simulink model "IntegratedLocalizationProcessor"  (R2023b)
settings: Solver=VariableStepAuto  StartTime=0.0  StopTime=10.0  RelTol=1e-3
undefined symbols (not defined in the file or in its folder): Discrete, fractalcoef, Time
libraries: mspsensorlib x1, ctrlSharedLib x1
settings Model: Creator=user  LastModifiedBy=user

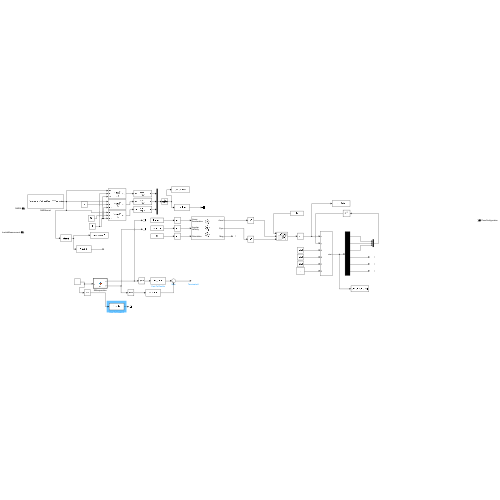
[thumbnail: Simulink's stored preview of the top-level diagram]
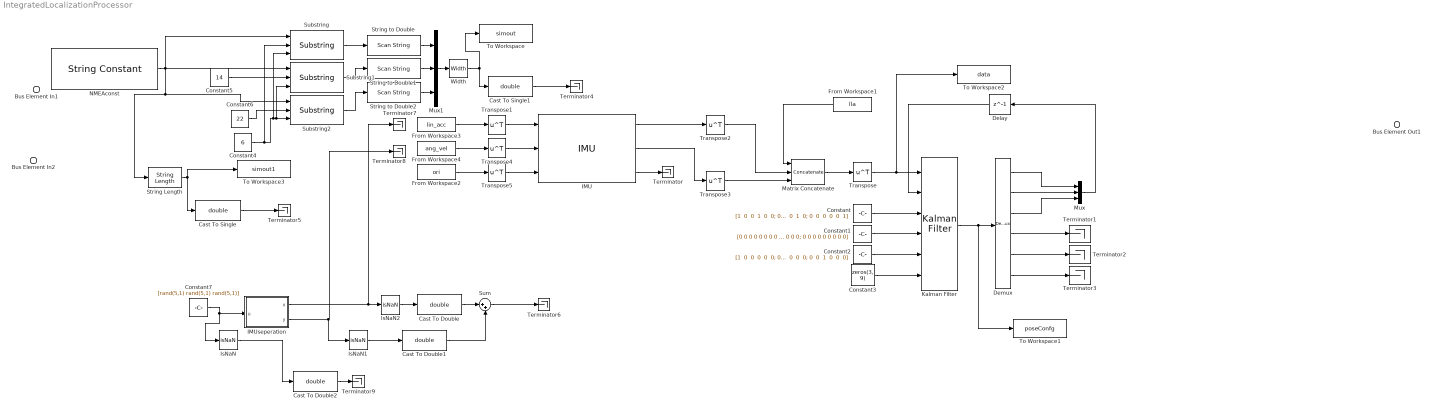
== system IntegratedLocalizationProcessor ==
  Bus Element In1 : Inport  PortName=NMEA
  Bus Element In2 : Inport  Port=2  PortName=InertialMeasurement
  Cast To Double : DataTypeConversion  OutDataTypeStr=double  SaturateOnIntegerOverflow=off  RndMeth=Floor
  Cast To Double1 : DataTypeConversion  OutDataTypeStr=double  SaturateOnIntegerOverflow=off  RndMeth=Floor
  Cast To Double2 : DataTypeConversion  OutDataTypeStr=double  SaturateOnIntegerOverflow=off  RndMeth=Floor
  Cast To Single : DataTypeConversion  OutDataTypeStr=double  SaturateOnIntegerOverflow=off  RndMeth=Floor
  Cast To Single1 : DataTypeConversion  OutDataTypeStr=double  SaturateOnIntegerOverflow=off  RndMeth=Floor
  Constant : Constant  Value=|
      | [1  0  0  1  0  0;
      | 0  1  0  0  1  0;
      | 0  0  1  0  0  1;
      | 0  0  0  1  0  0;
      | 0  0  0  0  1  0;
      | 0  0  0  0  0  1]
  Constant1 : Constant  Value=|
      | [0 0 0 0 0 0 0 0 0;
      | 0 0 0 0 0 0 0 0 0;
      | 0 0 0 0 0 0 0 0 0;
      | 0 0 0 0 0 0 0 0 0;
      | 0 0 0 0 0 0 0 0 0;
      | 0 0 0 0 0 0 0 0 0]
  Constant2 : Constant  Value="[1  0  0  0  0  0; 0  1  0  0  0  0; 0  0  1  0  0  0]"  VectorParams1D=off
  Constant3 : Constant  Value=zeros(3, 9)
  Constant4 : Constant  Value=6  OutDataTypeStr=uint16
  Constant5 : Constant  Value=14  OutDataTypeStr=uint8
  Constant6 : Constant  Value=22  OutDataTypeStr=uint8
  Constant7 : Constant  Value=[rand(5,1) rand(5,1) rand(5,1)]
  Delay : Delay  DelayLength=1
  Demux : Demux  Outputs=6
  From Workspace1 : FromWorkspace  VariableName=lla  SampleTime=1
  From Workspace2 : FromWorkspace  VariableName=ori  SampleTime=1
  From Workspace3 : FromWorkspace  VariableName=lin_acc  SampleTime=1
  From Workspace4 : FromWorkspace  VariableName=ang_vel  SampleTime=1
  IMU : mspsensorlib/IMU  DispRefFrame=NED  TemperaturePort=off  Temperature=25  MagneticFieldPort=off  MagneticFieldNED=[ 27.5550, -2.4169, -16.0849 ]  MagneticFieldENU=[ -2.4169, 27.5550, 16.0849 ]  SeedDouble=67  SimulateUsing=Interpreted execution  AccelParamsMeasurementRange=Inf  AccelParamsResolution=0  AccelParamsConstantBias=[ 0, 0, 0 ]  AccelParamsAxesMisalignment=[ 100, 0, 0; 0, 100, 0; 0, 0, 100 ]  AccelParamsNoiseDensity=[ 0, 0, 0 ]  AccelParamsBiasInstability=[ 0, 0, 0 ]  AccelParamsBiasInstabilityNumerator=fractalcoef().Numerator  AccelParamsBiasInstabilityDenominator=fractalcoef().Denominator  AccelParamsRandomWalk=[ 0, 0, 0 ]  AccelParamsNoiseType=double-sided  AccelParamsTemperatureBias=[ 0, 0, 0 ]  AccelParamsTemperatureScaleFactor=[ 0, 0, 0 ]  GyroParamsMeasurementRange=Inf  GyroParamsResolution=0  GyroParamsConstantBias=[ 0, 0, 0 ]  GyroParamsAxesMisalignment=[ 100, 0, 0; 0, 100, 0; 0, 0, 100 ]  GyroParamsAccelerationBias=[ 0, 0, 0 ]  GyroParamsNoiseDensity=[ 0, 0, 0 ]  GyroParamsBiasInstability=[ 0, 0, 0 ]  GyroParamsBiasInstabilityNumerator=fractalcoef().Numerator  GyroParamsBiasInstabilityDenominator=fractalcoef().Denominator  GyroParamsRandomWalk=[ 0, 0, 0 ]  GyroParamsNoiseType=double-sided  GyroParamsTemperatureBias=[ 0, 0, 0 ]  GyroParamsTemperatureScaleFactor=[ 0, 0, 0 ]  MagParamsMeasurementRange=Inf  MagParamsResolution=0  MagParamsConstantBias=[ 0, 0, 0 ]  MagParamsAxesMisalignment=[ 100, 0, 0; 0, 100, 0; 0, 0, 100 ]  MagParamsNoiseDensity=[ 0, 0, 0 ]  MagParamsBiasInstability=[ 0, 0, 0 ]  MagParamsBiasInstabilityNumerator=fractalcoef().Numerator  MagParamsBiasInstabilityDenominator=fractalcoef().Denominator  MagParamsRandomWalk=[ 0, 0, 0 ]  MagParamsNoiseType=double-sided  MagParamsTemperatureBias=[ 0, 0, 0 ]  MagParamsTemperatureScaleFactor=[ 0, 0, 0 ]
  IMUseperation : MATLAB Function  TreatAsAtomicUnit=on
  IsNaN : RelationalOperator  Operator=isNaN  OutDataTypeStr=boolean  RndMeth=Simplest  InputSameDT=off
  IsNaN1 : RelationalOperator  Operator=isNaN  OutDataTypeStr=boolean  RndMeth=Simplest  InputSameDT=off
  IsNaN2 : RelationalOperator  Operator=isNaN  OutDataTypeStr=boolean  RndMeth=Simplest  InputSameDT=off
  Kalman Filter : ctrlSharedLib/Kalman Filter  TimeDomain=Discrete-Time  UseCurrentEstimator=on  ModelSource=Input port  ModelSourceVariable=ss(0.95,1,1,0,1)  A=0.95  B=1  C=1  D=0  NumberOfStates=6  NumberOfInputs=9  NumberOfOutputs=3  InitialEstimateSource=Dialog  X0=0  P0=10  UseK=off  UseGH=off  NumberOfProcessNoiseInputs=1  G=1  TimeInvariantG=on  H=0  TimeInvariantH=on  Q=0.05  TimeInvariantQ=on  R=1  TimeInvariantR=on  N=0  TimeInvariantN=on  AddInputPort=on  AddEnablePort=off  OutputEstimatedY=off  OutputP=off  Ts=-1
  Matrix Concatenate : Concatenate  NumInputs=3  Mode=Multidimensional array
  Mux : Mux  Inputs=3
  Mux1 : Mux  Inputs=3
  NMEAconst : StringConstant  String="\"nmea,001400l,001600l,000001a,time12:33:12\""
  String Length : StringLength
  String to Double : ScanString  Format="\"%lf\""
  String to Double1 : ScanString  Format="\"%lf\""
  String to Double2 : ScanString  Format="\"%lf\""
  Substring : Substring
  Substring1 : Substring
  Substring2 : Substring
  Sum : Sum  Inputs=|++
  Terminator{,1..9} (10 alike) : Terminator
  To Workspace : ToWorkspace  VariableName=simout  SaveFormat=Timeseries  SampleTime=-1
  To Workspace1 : ToWorkspace  VariableName=poseConfg  SaveFormat=Timeseries  SampleTime=-1
  To Workspace2 : ToWorkspace  VariableName=data  SaveFormat=Timeseries  SampleTime=-1
  To Workspace3 : ToWorkspace  VariableName=simout1  SaveFormat=Timeseries  SampleTime=-1
  Transpose{,1..5} (6 alike) : Math  Operator=transpose
  Width : Width  DataType=uint8
  Bus Element Out1 : Outport  PortName=PoseConfiguration
  wires:
  Demux/5 -> Terminator2/1
  Demux/2 -> Mux/2
  Demux/1 -> Mux/1
  Mux/1 -> Delay/1
  Delay/1 -> Kalman Filter/2
  Kalman Filter/1 -> To Workspace1/1, Demux/1
  Demux/4 -> Terminator1/1
  Constant/1 -> Kalman Filter/3
  Demux/3 -> Mux/3
  Demux/6 -> Terminator3/1
  From Workspace3/1 -> Transpose1/1
  Constant3/1 -> Kalman Filter/6
  IMU/3 -> Terminator/1
  Transpose4/1 -> IMU/2
  Transpose3/1 -> Matrix Concatenate/3
  From Workspace4/1 -> Transpose4/1
  Transpose2/1 -> Matrix Concatenate/2
  From Workspace1/1 -> Matrix Concatenate/1
  Transpose5/1 -> IMU/3
  Constant1/1 -> Kalman Filter/4
  Matrix Concatenate/1 -> Transpose/1
  Transpose1/1 -> IMU/1
  Transpose/1 -> To Workspace2/1, Kalman Filter/1
  IMU/1 -> Transpose2/1
  IMU/2 -> Transpose3/1
  From Workspace2/1 -> Transpose5/1
  Constant2/1 -> Kalman Filter/5
  NMEAconst/1 -> Substring1/1, Substring/1, String Length/1, Substring2/1
  Mux1/1 -> Width/1
  Width/1 -> To Workspace/1, Cast To Single1/1
  String to Double/1 -> Mux1/1
  String to Double1/1 -> Mux1/2
  String to Double2/1 -> Mux1/3
  Substring/1 -> String to Double/1
  Substring1/1 -> String to Double1/1
  Substring2/1 -> String to Double2/1
  Constant4/1 -> Substring/2, Substring/3, Substring1/3, Substring2/3
  Constant5/1 -> Substring1/2
  Constant6/1 -> Substring2/2
  String Length/1 -> Cast To Single/1, To Workspace3/1
  Cast To Single/1 -> Terminator5/1
  Cast To Single1/1 -> Terminator4/1
  Constant7/1 -> IsNaN/1, IMUseperation/1(u)
  IsNaN/1 -> Cast To Double2/1
  IMUseperation/1(x) -> IsNaN2/1, Terminator7/1
  IMUseperation/2(y) -> IsNaN1/1, Terminator8/1
  IsNaN2/1 -> Cast To Double/1
  IsNaN1/1 -> Cast To Double1/1
  Sum/1 -> Terminator6/1
  Cast To Double/1 -> Sum/1
  Cast To Double1/1 -> Sum/2
  Cast To Double2/1 -> Terminator9/1

== matlab function IntegratedLocalizationProcessor/IMUseperation ==
  data: x output; u input; y output
function [x, y]= fcn(u)

x = zeros(3,1);
y = zeros(3,1);

x=u(1,:)';
y=u(1,:)';

end
